simulink model "massforce"  (R2018b)
settings: Solver=VariableStepAuto  StartTime=0.0  StopTime=10.0  RelTol=1e-3
settings Model: Creator=prakyath  LastModifiedBy=prakyath
settings DebuggingCC: LibraryContextMissingDiagnostic=none
settings SFSimCC: SimUseLocalCustomCode=off
settings RTWCC: RTWUseLocalCustomCode=off

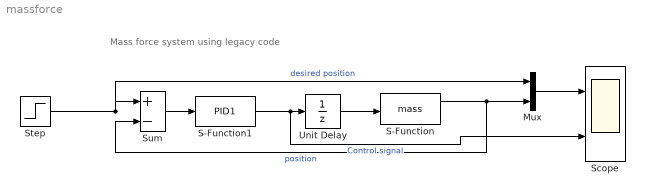
== system massforce ==
  note: Mass force system using legacy code
  Mux : Mux  Inputs=2
  "S-Function " : S-Function  FunctionName=mass  Parameters=0,5,1,0.001  SFunctionDeploymentMode=off  EnableBusSupport=off
  "S-Function1 " : S-Function  FunctionName=PID1  Parameters=25,0,5  SFunctionDeploymentMode=off  EnableBusSupport=off
  Scope : Scope  NumInputPorts=2
  Step : Step  SampleTime=0
  Sum : Sum  Inputs=|+-
  Unit Delay : UnitDelay  SampleTime=0.001
  wires:
  Unit Delay/1 -> "S-Function "/1
  "S-Function1 "/1 -> Scope/2, Unit Delay/1  "Control signal"
  Sum/1 -> "S-Function1 "/1
  Step/1 -> Mux/1, Sum/1  "desired position"
  "S-Function "/1 -> Mux/2, Sum/2  "position"
  Mux/1 -> Scope/1
